simulink model "SMC_PC_Quadcopter_Simulation_SPC_ver2"  (R2013b)
settings: Solver=ode4  StartTime=0.0  StopTime=25  FixedStep=0.02  MaxStep=0.06  RelTol=1e-3
model workspace (MAT data in the model file):
  Sig = Simulink.Signal
  Sig.DataType = 'auto'
  Sig.Dimensions = -1
  Sig.DimensionsMode = 'auto'
  Sig.Complexity = 'auto'
  Sig.SampleTime = -1
  Sig.SamplingMode = 'auto'
undefined symbols (not defined in the file): IC, quadModel
Description:
  | This is a configurable quadcopter simulation.
  | This Simulink model demonstates position control.
  | 
  | Additional quadcopter modeling and simulation materials available at:
  | github.com/dch33/Quad-Sim
  | 
  | Copyright (C) 2014 D. Hartman, K. Landis, S. Moreno, J. Kim, M. Mehrer
  | 
  | License:
  |     This program is free software: you can redistribute it and/or modify
  |     it under the terms of the GNU LESSER GENERAL PUBLIC LICENSE as published by
  |     the Free Software Foundation, either version 3 of the License, or
  |     (at your option) any later version.
  | 
  |     This program is distributed in the hope that it will be useful,
  |     but WITHOUT ANY WARRANTY; without even the implied warranty of
  |     MERCHANTABILITY or FITNESS FOR A PARTICULAR PURPOSE.  See the
  |     GNU General Public License for more details.
  | 
  |     You should have received a copy of the GNU LESSER GENERAL PUBLIC LICENSE
  |     along with this program.  If not, see <http://www.gnu.org/licenses/>.
settings Model: ModifiedComment=SwiftWind -- Mon Apr 06 22:59:35 2015 -- Version 1.6  Creator=David Hartman  LastModifiedBy=SwiftWind
settings Model: ModifiedHistory=|
  | SwiftWind -- Mon Apr 06 22:59:35 2015 -- Version 1.6
  | 
  | 
  | SwiftWind -- Mon Apr 06 22:59:35 2015 -- Version 1.6
  | 
  | 
  | davidhartman -- Fri Jun 06 22:59:54 2014 -- Version 1.5
settings DataIOCC: LimitDataPoints=off  SignalLogging=off
settings OptimizationCC: InlineParams=on
settings DebuggingCC: UnderspecifiedInitializationDetection=Simplified  MergeDetectMultiDrivingBlocksExec=error  UniqueDataStoreMsg=warning  StateNameClashWarn=warning  StrictBusMsg=ErrorOnBusTreatedAsVector

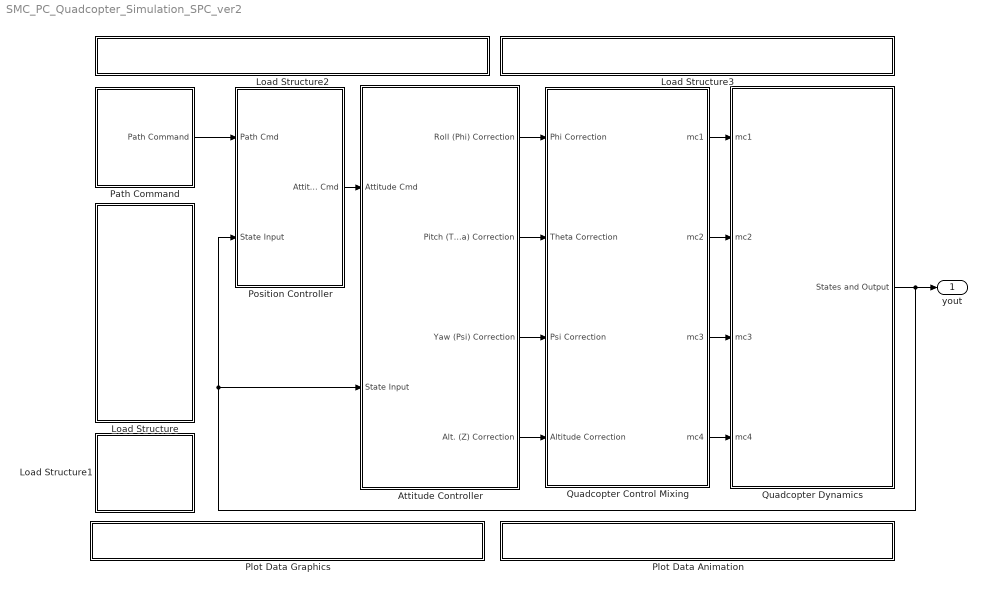
== system SMC_PC_Quadcopter_Simulation_SPC_ver2 ==
  Attitude Controller : Subsystem
  Load Structure : Subsystem
      settings: OpenFcn=|
      | uiopen('load')
      | if ((exist('IC')==1) && (exist('quadModel')==1) && (exist('path')==1))
      | set_param(bdroot, 'SimulationCommand', 'update')
      | end
      mask Display: fprintf('LOAD:\nTimeseries\nPath\nCommands,\nQuadcopter\nModel, Or\nInitial\nConditions');
  Load Structure1 : Subsystem
      settings: OpenFcn=|
      | if (exist('IC')==1 && exist('quadModel')==1 && exist('yout') && exist('tout'))
      | saveSimResults()
      | else
      | msgbox('No Data To Save!')
      | end
      mask Display: fprintf('SAVE:\nSimulation\nResults');
  Load Structure2 : Subsystem
      settings: OpenFcn=|
      | if exist('GUI_Modeling') == 2,
      | run('GUI_Modeling')
      | 
      | else
      | 
      | msgbox('The desired GUI must be first added to MATLABs path.')
      | 
      | end
      mask Display: fprintf('OPEN GUI: Build New \n Model');
  Load Structure3 : Subsystem
      settings: OpenFcn=|
      | if exist('GUI_IC') == 2,
      | run('GUI_IC')
      | 
      | else
      | 
      | msgbox('The desired GUI must be first added to MATLABs path.')
      | 
      | end
      mask Display: fprintf('OPEN GUI: Create Initial \n Conditions');
  Path Command : Subsystem  mask{Interpolate=on, OutputAfterFinalValue=Holding final value}
      mask prompts: Interpolate "Interpolate X, Y, Z, and Psi command data?"; OutputAfterFinalValue "Form output after final data value by:"
      mask help:
      | Selecting the Interpolate data checkbox causes position commands to be
      | linearly interpolated. For additional options related to the Timeseries
      | "path" commands, look under the block and click on the Timeseries From
      | Workspace blocks.
      mask TypeOptions Interpolate: X Timeseries From Wkspace/Interpolate | Y Timeseries From Wkspace/Interpolate | Z Timeseries From Wkspace/Interpolate | Psi Timeseries From Wkspace/Interpolate
      mask TypeOptions OutputAfterFinalValue: X Timeseries From Wkspace/OutputAfterFinalValue | Y Timeseries From Wkspace/OutputAfterFinalValue | Z Timeseries From Wkspace/OutputAfterFinalValue | Psi Timeseries From Wkspace/OutputAfterFinalValue
  Plot Data Animation : Subsystem
      settings: OpenFcn=|
      | if exist('QuadAnim4') == 2,
      |     if exist('yout')
      | 	run('QuadAnim4');
      |     else
      |     msgbox('Simulation must be run before data can be plotted.');
      |     end
      | else                                                                          msgbox('The desired GUI must be first added to MATLABs path.')
      | end
      mask Display: fprintf('OPEN GUI: Flight Animation')
  Plot Data Graphics : Subsystem
      settings: OpenFcn=|
      | if exist('yout')
      | yout = evalin('base', 'yout');
      | tout = evalin('base', 'tout');
      | quadPlots(yout, tout)
      | else
      | msgbox('Simulation must be run before data can be plotted.')
      | end
      mask Display: fprintf('OPEN PLOT: State Data')
  Position Controller : Subsystem
  Quadcopter Control Mixing : Subsystem
      mask Display:
      | modelLoaded = evalin('base','exist(''quadModel'',''var'')');
      | if (modelLoaded==1)
      |     if (evalin('base','quadModel.plusConfig'))
      |     fprintf([' \n' ' \n'  'Configuration "+"']);
      |     else if (~evalin('base','quadModel.plusConfig'))
      |         fprintf([' \n' ' \n' 'Configuration "X"']);
      |         end
      |     end
      | else
      |     fprintf([' \n' ' \n'  'Model Not Loaded']);
      | end
  Quadcopter Dynamics : Subsystem
  yout : Outport
  wires:
  Quadcopter Control Mixing/1(mc1) -> Quadcopter Dynamics/1(mc1)
  Quadcopter Control Mixing/2(mc2) -> Quadcopter Dynamics/2(mc2)
  Quadcopter Control Mixing/3(mc3) -> Quadcopter Dynamics/3(mc3)
  Quadcopter Control Mixing/4(mc4) -> Quadcopter Dynamics/4(mc4)
  Quadcopter Dynamics/1(States and Output) -> yout/1, Attitude Controller/2(State Input), Position Controller/2(State Input)
  Attitude Controller/1(Roll (Phi) Correction) -> Quadcopter Control Mixing/1(Phi Correction)
  Attitude Controller/2(Pitch (Theta) Correction) -> Quadcopter Control Mixing/2(Theta Correction)
  Attitude Controller/3(Yaw (Psi) Correction) -> Quadcopter Control Mixing/3(Psi Correction)
  Attitude Controller/4(Alt. (Z) Correction) -> Quadcopter Control Mixing/4(Altitude Correction)
  Path Command/1("Path Command ") -> Position Controller/1(Path Cmd)
  Position Controller/1(Attitude Cmd) -> Attitude Controller/1(Attitude Cmd)

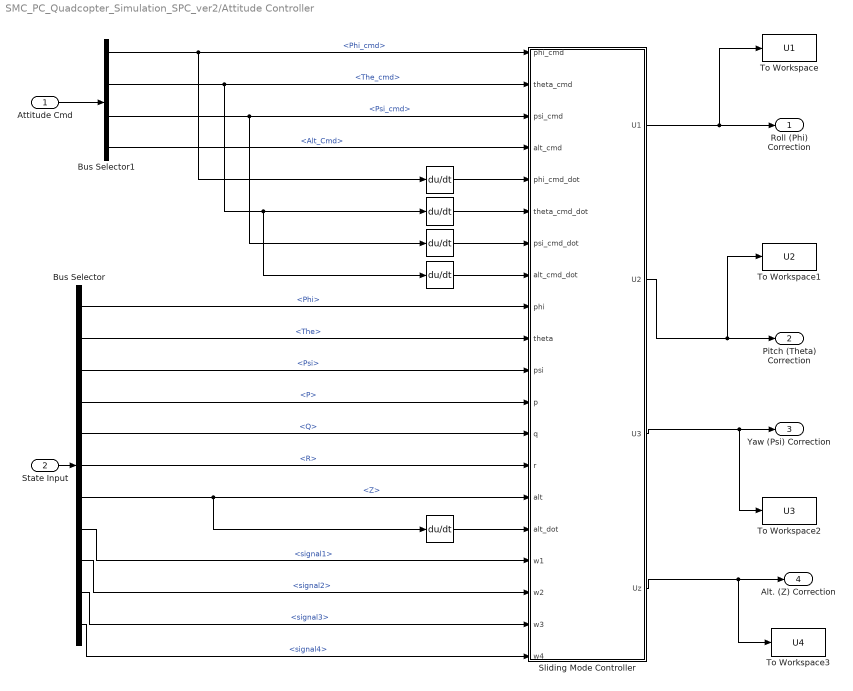
== system SMC_PC_Quadcopter_Simulation_SPC_ver2/Attitude Controller ==
  Attitude Cmd : Inport
  State Input : Inport  Port=2
  " " : Derivative
  " " : Derivative
  "    " : Derivative
  "      " : Derivative
  "        " : Derivative
  Bus Selector : BusSelector  OutputSignals=Phi,The,Psi,P,Q,R,Z,mc and RPM.signal1,mc and RPM.signal2,mc and RPM.signal3,mc and RPM.signal4
  Bus Selector1 : BusSelector  OutputSignals=Phi_cmd,The_cmd,Psi_cmd,Alt_Cmd
  Sliding Mode Controller : MATLAB Function  TreatAsAtomicUnit=on
  To Workspace : ToWorkspace  VariableName=U1  SampleTime=-1  SaveFormat=Timeseries
  To Workspace1 : ToWorkspace  VariableName=U2  SampleTime=-1  SaveFormat=Timeseries
  To Workspace2 : ToWorkspace  VariableName=U3  SampleTime=-1  SaveFormat=Timeseries
  To Workspace3 : ToWorkspace  VariableName=U4  SampleTime=-1  SaveFormat=Timeseries
  Roll (Phi) Correction : Outport
  Pitch (Theta) Correction : Outport  Port=2
  Yaw (Psi) Correction : Outport  Port=3
  Alt. (Z) Correction : Outport  Port=4
  wires:
  Bus Selector/6 -> Sliding Mode Controller/14(r)  "<R>"
  Bus Selector/5 -> Sliding Mode Controller/13(q)  "<Q>"
  Bus Selector/2 -> Sliding Mode Controller/10(theta)  "<The>"
  Bus Selector/3 -> Sliding Mode Controller/11(psi)  "<Psi>"
  State Input/1 -> Bus Selector/1
  Bus Selector/8 -> Sliding Mode Controller/17(w1)  "<signal1>"
  Bus Selector/9 -> Sliding Mode Controller/18(w2)  "<signal2>"
  Bus Selector/10 -> Sliding Mode Controller/19(w3)  "<signal3>"
  Bus Selector/11 -> Sliding Mode Controller/20(w4)  "<signal4>"
  Bus Selector/1 -> Sliding Mode Controller/9(phi)  "<Phi>"
  Bus Selector/7 -> Sliding Mode Controller/15(alt), "        "/1  "<Z>"
  Bus Selector/4 -> Sliding Mode Controller/12(p)  "<P>"
  Attitude Cmd/1 -> Bus Selector1/1
  Bus Selector1/1 -> Sliding Mode Controller/1(phi_cmd), " "/1  "<Phi_cmd>"
  Bus Selector1/2 -> " "/1, "      "/1, Sliding Mode Controller/2(theta_cmd)  "<The_cmd>"
  Bus Selector1/3 -> "    "/1, Sliding Mode Controller/3(psi_cmd)  "<Psi_cmd>"
  Bus Selector1/4 -> Sliding Mode Controller/4(alt_cmd)  "<Alt_Cmd>"
  " "/1 -> Sliding Mode Controller/5(phi_cmd_dot)
  " "/1 -> Sliding Mode Controller/6(theta_cmd_dot)
  "    "/1 -> Sliding Mode Controller/7(psi_cmd_dot)
  "      "/1 -> Sliding Mode Controller/8(alt_cmd_dot)
  Sliding Mode Controller/4(Uz) -> To Workspace3/1, Alt. (Z) Correction/1
  Sliding Mode Controller/1(U1) -> To Workspace/1, Roll (Phi) Correction/1
  Sliding Mode Controller/2(U2) -> To Workspace1/1, Pitch (Theta) Correction/1
  Sliding Mode Controller/3(U3) -> Yaw (Psi) Correction/1, To Workspace2/1
  "        "/1 -> Sliding Mode Controller/16(alt_dot)

== system SMC_PC_Quadcopter_Simulation_SPC_ver2/Load Structure ==

== system SMC_PC_Quadcopter_Simulation_SPC_ver2/Load Structure1 ==

== system SMC_PC_Quadcopter_Simulation_SPC_ver2/Load Structure2 ==

== system SMC_PC_Quadcopter_Simulation_SPC_ver2/Load Structure3 ==

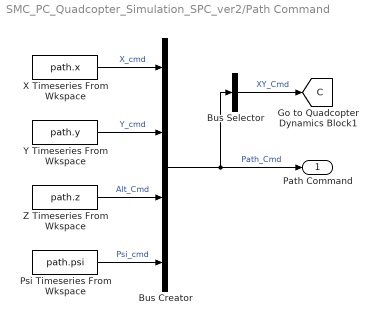
== system SMC_PC_Quadcopter_Simulation_SPC_ver2/Path Command ==
  Bus Creator : BusCreator
  Bus Selector : BusSelector  OutputSignals=X_cmd,Y_cmd  OutputAsBus=on
  Psi Timeseries From Wkspace : FromWorkspace  VariableName=path.psi  SampleTime=0  OutputAfterFinalValue=Holding final value
  X Timeseries From Wkspace : FromWorkspace  VariableName=path.x  SampleTime=0  OutputAfterFinalValue=Holding final value
  Y Timeseries From Wkspace : FromWorkspace  VariableName=path.y  SampleTime=0  OutputAfterFinalValue=Holding final value
  Z Timeseries From Wkspace : FromWorkspace  VariableName=path.z  SampleTime=0  OutputAfterFinalValue=Holding final value
  "Path Command " : Outport
  tag scope: C=global
  wires:
  X Timeseries From Wkspace/1 -> Bus Creator/1  "X_cmd"
  Y Timeseries From Wkspace/1 -> Bus Creator/2  "Y_cmd"
  Z Timeseries From Wkspace/1 -> Bus Creator/3  "Alt_Cmd"
  Psi Timeseries From Wkspace/1 -> Bus Creator/4  "Psi_cmd"
  Bus Creator/1 -> Bus Selector/1, "Path Command "/1  "Path_Cmd"
  Bus Selector/1 -> [C]  "XY_Cmd"

== system SMC_PC_Quadcopter_Simulation_SPC_ver2/Plot Data Animation ==

== system SMC_PC_Quadcopter_Simulation_SPC_ver2/Plot Data Graphics ==

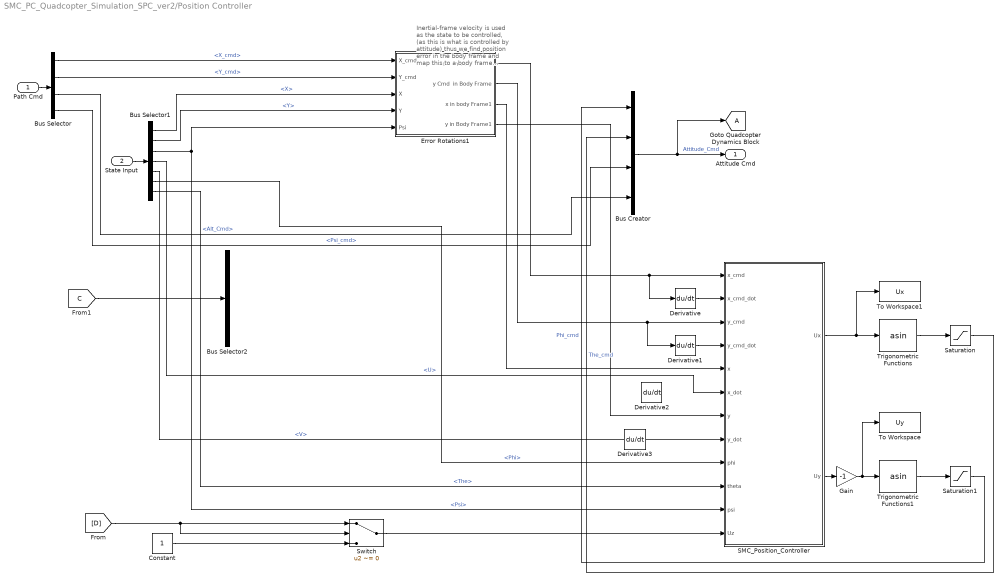
== system SMC_PC_Quadcopter_Simulation_SPC_ver2/Position Controller ==
  note: Inertial-frame velocity is used as the state to be controlled,
      | (as this is what is controlled by attitude)
      | thus we find position error in the body frame
      | and map this to a body frame desired velocity. This desired
      | velocity is then mapped to a desired attitude.
  Path Cmd : Inport
  State Input : Inport  Port=2
  Bus Creator : BusCreator
  Bus Selector : BusSelector  OutputSignals=X_cmd,Y_cmd,Alt_Cmd,Psi_cmd
  Bus Selector1 : BusSelector  OutputSignals=X,Y,Psi,U,V,Phi,The
  Bus Selector2 : BusSelector  OutputSignals=X_cmd,Y_cmd
  Constant : Constant
  Derivative{,1..3} (4 alike) : Derivative
  Error Rotations1 : Subsystem
  Gain : Gain  Gain=-1
  SMC_Position_Controller : MATLAB Function  TreatAsAtomicUnit=on
  Saturation : Saturate  UpperLimit=20*pi/180  LowerLimit=-20*pi/180
  Saturation1 : Saturate  UpperLimit=20*pi/180  LowerLimit=-20*pi/180
  Switch : Switch  Criteria=u2 ~= 0
  To Workspace : ToWorkspace  VariableName=Uy  SampleTime=-1  SaveFormat=Timeseries
  To Workspace1 : ToWorkspace  VariableName=Ux  SampleTime=-1  SaveFormat=Timeseries
  Trigonometric Functions : Trigonometry  Operator=asin
  Trigonometric Functions1 : Trigonometry  Operator=asin
  Attitude Cmd : Outport
  tag scope: A=global
  wires:
  Bus Selector1/5 -> SMC_Position_Controller/8(y_dot)  "<V>"
  State Input/1 -> Bus Selector1/1
  Bus Selector/4 -> Bus Creator/3  "<Psi_cmd>"
  Path Cmd/1 -> Bus Selector/1
  Bus Selector/3 -> Bus Creator/4  "<Alt_Cmd>"
  Bus Creator/1 -> Attitude Cmd/1, [A]  "Attitude_Cmd"
  Bus Selector/1 -> Error Rotations1/1(X_cmd)  "<X_cmd>"
  Bus Selector/2 -> Error Rotations1/2(Y_cmd)  "<Y_cmd>"
  Bus Selector1/1 -> Error Rotations1/3(X)  "<X>"
  Bus Selector1/2 -> Error Rotations1/4(Y)  "<Y>"
  Bus Selector1/3 -> Error Rotations1/5(Psi), SMC_Position_Controller/11(psi)  "<Psi>"
  Bus Selector1/4 -> SMC_Position_Controller/6(x_dot)  "<U>"
  [C] -> Bus Selector2/1
  Derivative/1 -> SMC_Position_Controller/2(x_cmd_dot)
  Derivative1/1 -> SMC_Position_Controller/4(y_cmd_dot)
  Bus Selector1/6 -> SMC_Position_Controller/9(phi)  "<Phi>"
  Bus Selector1/7 -> SMC_Position_Controller/10(theta)  "<The>"
  SMC_Position_Controller/1(Ux) -> To Workspace1/1, Trigonometric Functions/1
  [D] -> Switch/2, Switch/1
  Constant/1 -> Switch/3
  Switch/1 -> SMC_Position_Controller/12(Uz)
  Trigonometric Functions/1 -> Saturation/1
  Trigonometric Functions1/1 -> Saturation1/1
  Saturation1/1 -> Bus Creator/1  "Phi_cmd"
  Saturation/1 -> Bus Creator/2  "The_cmd"
  Error Rotations1/1(x Cmd  in body Frame) -> Derivative/1, SMC_Position_Controller/1(x_cmd)
  Error Rotations1/2(y Cmd  in Body Frame) -> Derivative1/1, SMC_Position_Controller/3(y_cmd)
  Error Rotations1/3(x in body Frame1) -> SMC_Position_Controller/5(x)
  Error Rotations1/4(y in Body Frame1) -> SMC_Position_Controller/7(y)
  SMC_Position_Controller/2(Uy) -> Gain/1
  Gain/1 -> To Workspace/1, Trigonometric Functions1/1

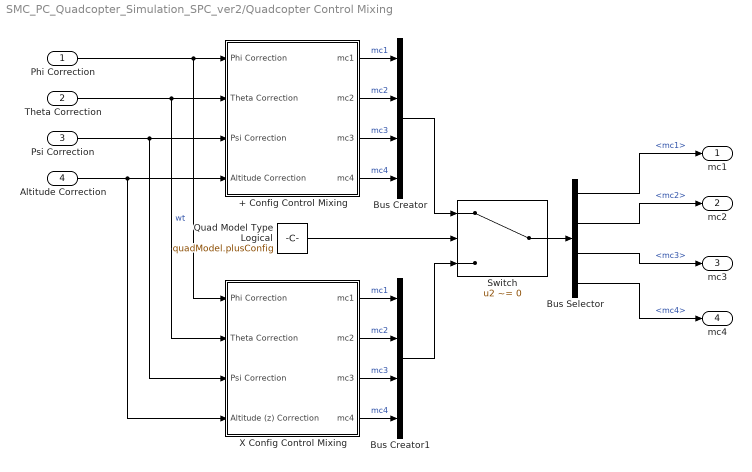
== system SMC_PC_Quadcopter_Simulation_SPC_ver2/Quadcopter Control Mixing ==
  Phi Correction : Inport
  Theta Correction : Inport  Port=2
  Psi Correction : Inport  Port=3
  Altitude Correction : Inport  Port=4
  + Config Control Mixing : Subsystem
  Bus Creator : BusCreator
  Bus Creator1 : BusCreator
  Bus Selector : BusSelector  OutputSignals=mc1,mc2,mc3,mc4
  Quad Model Type Logical : Constant  Value=quadModel.plusConfig
  Switch : Switch  Criteria=u2 ~= 0
  X Config Control Mixing : Subsystem
  mc1 : Outport
  mc2 : Outport  Port=2
  mc3 : Outport  Port=3
  mc4 : Outport  Port=4
  wires:
  Phi Correction/1 -> X Config Control Mixing/1(Phi Correction), + Config Control Mixing/1(Phi Correction)
  Theta Correction/1 -> X Config Control Mixing/2(Theta Correction), + Config Control Mixing/2(Theta Correction)  "wt"
  Psi Correction/1 -> X Config Control Mixing/3(Psi Correction), + Config Control Mixing/3(Psi Correction)
  Altitude Correction/1 -> X Config Control Mixing/4(Altitude (z) Correction), + Config Control Mixing/4(Altitude Correction)
  + Config Control Mixing/1(mc1) -> Bus Creator/1  "mc1"
  + Config Control Mixing/2(mc2) -> Bus Creator/2  "mc2"
  + Config Control Mixing/3(mc3) -> Bus Creator/3  "mc3"
  + Config Control Mixing/4(mc4) -> Bus Creator/4  "mc4"
  Bus Creator/1 -> Switch/1
  X Config Control Mixing/1(mc1) -> Bus Creator1/1  "mc1"
  X Config Control Mixing/2(mc2) -> Bus Creator1/2  "mc2"
  X Config Control Mixing/3(mc3) -> Bus Creator1/3  "mc3"
  X Config Control Mixing/4(mc4) -> Bus Creator1/4  "mc4"
  Bus Creator1/1 -> Switch/3
  Bus Selector/1 -> mc1/1  "<mc1>"
  Bus Selector/2 -> mc2/1  "<mc2>"
  Bus Selector/3 -> mc3/1  "<mc3>"
  Bus Selector/4 -> mc4/1  "<mc4>"
  Quad Model Type Logical/1 -> Switch/2
  Switch/1 -> Bus Selector/1

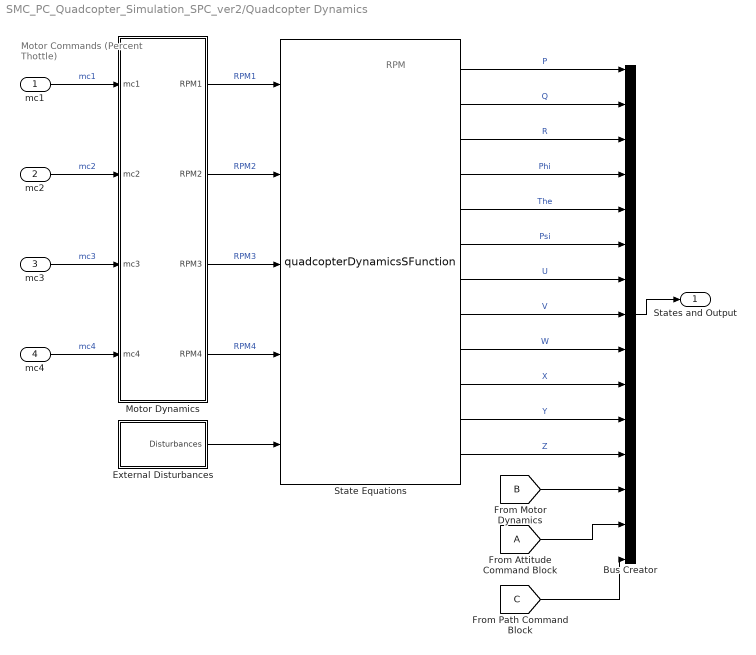
== system SMC_PC_Quadcopter_Simulation_SPC_ver2/Quadcopter Dynamics ==
  note: RPM
  note: Motor Commands
      | (Percent Thottle)
  mc1 : Inport
  mc2 : Inport  Port=2
  mc3 : Inport  Port=3
  mc4 : Inport  Port=4
  Bus Creator : BusCreator  Inputs='P','Q','R','Phi','The','Psi','U','V','W','X','Y','Z','mc and RPM','Attitude_Cmd','XY_Cmd'
  External Disturbances : Subsystem
  Motor Dynamics : Subsystem
  State Equations : M-S-Function  FunctionName=quadcopterDynamicsSFunction  Parameters=quadModel, IC
      mask Display:
      | port_label('input', 1, 'RPM1')
      | port_label('input', 2, 'RPM2')
      | port_label('input', 3, 'RPM3')
      | port_label('input', 4, 'RPM4')
      | port_label('input', 5, 'Disturbances')
      | port_label('output', 1, 'P')
      | port_label('output', 2, 'Q')
      | port_label('output', 3, 'R')
      | port_label('output', 4, 'Phi')
      | port_label('output', 5, 'The')
      | port_label('output', 6, 'Psi')
      | port_label('output', 7, 'U')
      | port_label('output', 8, 'V')
      | port_label('output', 9, 'W')
      | port_label('output', 10, 'X')
      | port_label('output', 11, 'Y')
      | port_label('output', 12, 'Z')
  States and Output : Outport
  wires:
  State Equations/1 -> Bus Creator/1  "P"
  State Equations/2 -> Bus Creator/2  "Q"
  State Equations/3 -> Bus Creator/3  "R"
  State Equations/4 -> Bus Creator/4  "Phi"
  State Equations/5 -> Bus Creator/5  "The"
  State Equations/6 -> Bus Creator/6  "Psi"
  State Equations/7 -> Bus Creator/7  "U"
  State Equations/8 -> Bus Creator/8  "V"
  State Equations/9 -> Bus Creator/9  "W"
  State Equations/10 -> Bus Creator/10  "X"
  State Equations/11 -> Bus Creator/11  "Y"
  State Equations/12 -> Bus Creator/12  "Z"
  Bus Creator/1 -> States and Output/1
  Motor Dynamics/1(RPM1) -> State Equations/1  "RPM1"
  Motor Dynamics/2(RPM2) -> State Equations/2  "RPM2"
  Motor Dynamics/3(RPM3) -> State Equations/3  "RPM3"
  Motor Dynamics/4(RPM4) -> State Equations/4  "RPM4"
  mc1/1 -> Motor Dynamics/1(mc1)  "mc1"
  mc4/1 -> Motor Dynamics/4(mc4)  "mc4"
  mc3/1 -> Motor Dynamics/3(mc3)  "mc3"
  mc2/1 -> Motor Dynamics/2(mc2)  "mc2"
  External Disturbances/1("Disturbances ") -> State Equations/5
  [A] -> Bus Creator/14
  [B] -> Bus Creator/13
  [C] -> Bus Creator/15

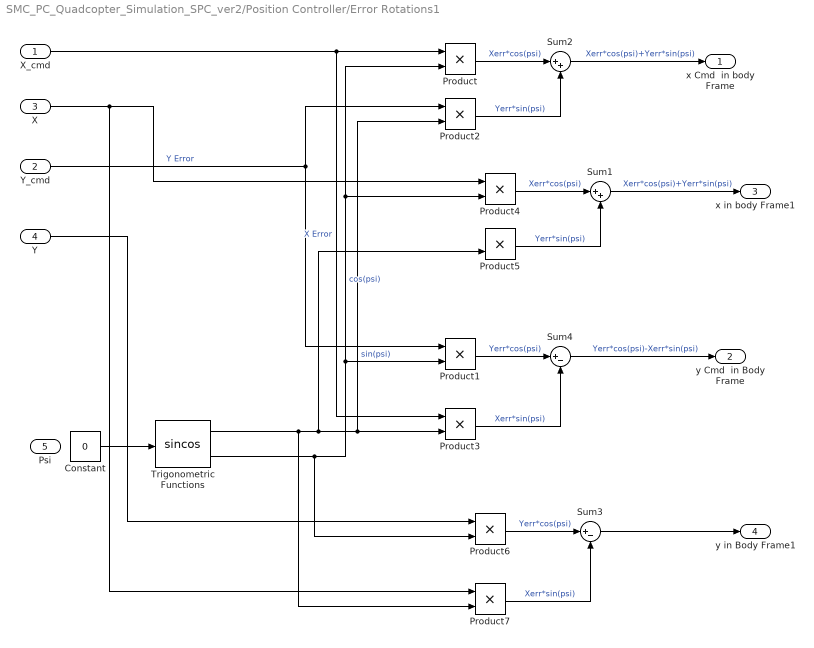
== system SMC_PC_Quadcopter_Simulation_SPC_ver2/Position Controller/Error Rotations1 ==
  X_cmd : Inport
  Y_cmd : Inport  Port=2
  X : Inport  Port=3
  Y : Inport  Port=4
  Psi : Inport  Port=5
  Constant : Constant  Value=0
  Product{,1..7} (8 alike) : Product
  Sum1 : Sum  Inputs=|++
  Sum2 : Sum  Inputs=|++
  Sum3 : Sum  Inputs=|+-
  Sum4 : Sum  Inputs=|+-
  Trigonometric Functions : Trigonometry  Operator=sincos
  x Cmd  in body Frame : Outport
  y Cmd  in Body Frame : Outport  Port=2
  x in body Frame1 : Outport  Port=3
  y in Body Frame1 : Outport  Port=4
  wires:
  Product1/1 -> Sum4/1  "Yerr*cos(psi)"
  Product2/1 -> Sum2/2  "Yerr*sin(psi)"
  Product/1 -> Sum2/1  "Xerr*cos(psi)"
  Trigonometric Functions/2 -> Product6/2, Product1/2, Product/2, Product4/2  "cos(psi)"
  X_cmd/1 -> Product/1, Product3/1  "X Error"
  Y/1 -> Product6/1
  Sum2/1 -> x Cmd  in body Frame/1  "Xerr*cos(psi)+Yerr*sin(psi)"
  Trigonometric Functions/1 -> Product7/2, Product5/2, Product3/2, Product2/2  "sin(psi)"
  Y_cmd/1 -> Product1/1, Product2/1  "Y Error"
  Product3/1 -> Sum4/2  "Xerr*sin(psi)"
  Sum4/1 -> y Cmd  in Body Frame/1  "Yerr*cos(psi)-Xerr*sin(psi)"
  Product5/1 -> Sum1/2  "Yerr*sin(psi)"
  Product4/1 -> Sum1/1  "Xerr*cos(psi)"
  Sum1/1 -> x in body Frame1/1  "Xerr*cos(psi)+Yerr*sin(psi)"
  X/1 -> Product7/1, Product4/1
  Product6/1 -> Sum3/1  "Yerr*cos(psi)"
  Product7/1 -> Sum3/2  "Xerr*sin(psi)"
  Sum3/1 -> y in Body Frame1/1
  Constant/1 -> Trigonometric Functions/1

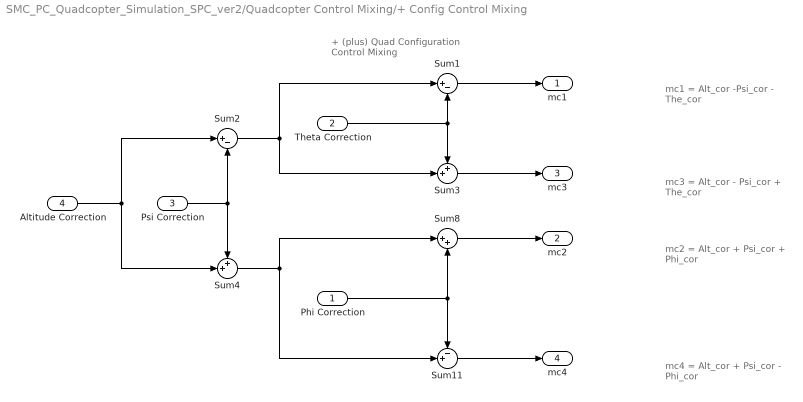
== system SMC_PC_Quadcopter_Simulation_SPC_ver2/Quadcopter Control Mixing/+ Config Control Mixing ==
  note: mc2 = Alt_cor + Psi_cor + Phi_cor
  note: + (plus) Quad Configuration Control Mixing
  note: mc4 = Alt_cor + Psi_cor - Phi_cor
  note: mc3 = Alt_cor - Psi_cor + The_cor
  note: mc1 = Alt_cor -Psi_cor - The_cor
  Phi Correction : Inport
  Theta Correction : Inport  Port=2
  Psi Correction : Inport  Port=3
  Altitude Correction : Inport  Port=4
  Sum1 : Sum  Inputs=|+-
  Sum11 : Sum  Inputs=-+|
  Sum2 : Sum  Inputs=|+-
  Sum3 : Sum  Inputs=++|
  Sum4 : Sum  Inputs=++|
  Sum8 : Sum  Inputs=|++
  mc1 : Outport
  mc2 : Outport  Port=2
  mc3 : Outport  Port=3
  mc4 : Outport  Port=4
  wires:
  Theta Correction/1 -> Sum1/2, Sum3/1
  Altitude Correction/1 -> Sum2/1, Sum4/2
  Sum2/1 -> Sum3/2, Sum1/1
  Psi Correction/1 -> Sum4/1, Sum2/2
  Sum4/1 -> Sum11/2, Sum8/1
  Phi Correction/1 -> Sum8/2, Sum11/1
  Sum1/1 -> mc1/1
  Sum3/1 -> mc3/1
  Sum8/1 -> mc2/1
  Sum11/1 -> mc4/1

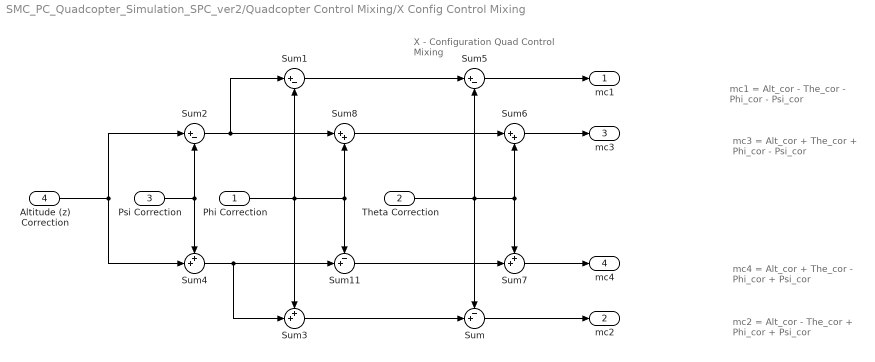
== system SMC_PC_Quadcopter_Simulation_SPC_ver2/Quadcopter Control Mixing/X Config Control Mixing ==
  note: mc1 = Alt_cor - The_cor - Phi_cor - Psi_cor
  note: X - Configuration Quad Control Mixing
  note: mc3 = Alt_cor + The_cor + Phi_cor - Psi_cor
  note: mc2 = Alt_cor - The_cor + Phi_cor + Psi_cor
  note: mc4 = Alt_cor + The_cor - Phi_cor + Psi_cor
  Phi Correction : Inport
  Theta Correction : Inport  Port=2
  Psi Correction : Inport  Port=3
  Altitude (z) Correction : Inport  Port=4
  Sum : Sum  Inputs=-+|
  Sum1 : Sum  Inputs=|+-
  Sum11 : Sum  Inputs=-+|
  Sum2 : Sum  Inputs=|+-
  Sum3 : Sum  Inputs=++|
  Sum4 : Sum  Inputs=++|
  Sum5 : Sum  Inputs=|+-
  Sum6 : Sum  Inputs=|++
  Sum7 : Sum  Inputs=++|
  Sum8 : Sum  Inputs=|++
  mc1 : Outport
  mc2 : Outport  Port=2
  mc3 : Outport  Port=3
  mc4 : Outport  Port=4
  wires:
  Sum2/1 -> Sum8/1, Sum1/1
  Psi Correction/1 -> Sum4/1, Sum2/2
  Phi Correction/1 -> Sum3/1, Sum1/2, Sum8/2, Sum11/1
  Sum4/1 -> Sum3/2, Sum11/2
  Sum3/1 -> Sum/2
  Theta Correction/1 -> Sum7/1, Sum6/2, Sum5/2, Sum/1
  Sum1/1 -> Sum5/1
  Sum8/1 -> Sum6/1
  Sum11/1 -> Sum7/2
  Sum5/1 -> mc1/1
  Sum6/1 -> mc3/1
  Sum7/1 -> mc4/1
  Altitude (z) Correction/1 -> Sum2/1, Sum4/2
  Sum/1 -> mc2/1

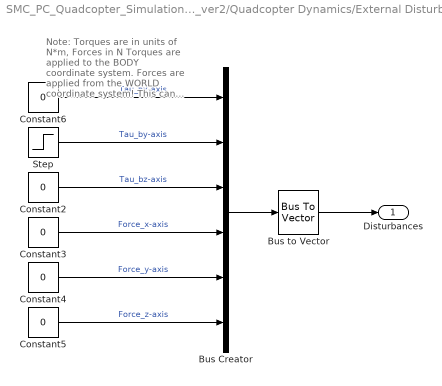
== system SMC_PC_Quadcopter_Simulation_SPC_ver2/Quadcopter Dynamics/External Disturbances ==
  note: Note: Torques are in units of N*m, Forces in N
      | Torques are applied to the BODY coordinate system.
      | Forces are applied from the WORLD coordinate system!
      | This can be changed by adjusting the equations within the S-function.
  Bus Creator : BusCreator  Inputs=6
  Bus to Vector : BusToVector
  Constant{2..6} (5 alike) : Constant  Value=0
  Step : Step  After=0  SampleTime=0
  "Disturbances " : Outport
  wires:
  Bus to Vector/1 -> "Disturbances "/1
  Bus Creator/1 -> Bus to Vector/1
  Constant6/1 -> Bus Creator/1  "Tau_bx-axis"
  Step/1 -> Bus Creator/2  "Tau_by-axis"
  Constant2/1 -> Bus Creator/3  "Tau_bz-axis"
  Constant3/1 -> Bus Creator/4  "Force_x-axis"
  Constant4/1 -> Bus Creator/5  "Force_y-axis"
  Constant5/1 -> Bus Creator/6  "Force_z-axis"

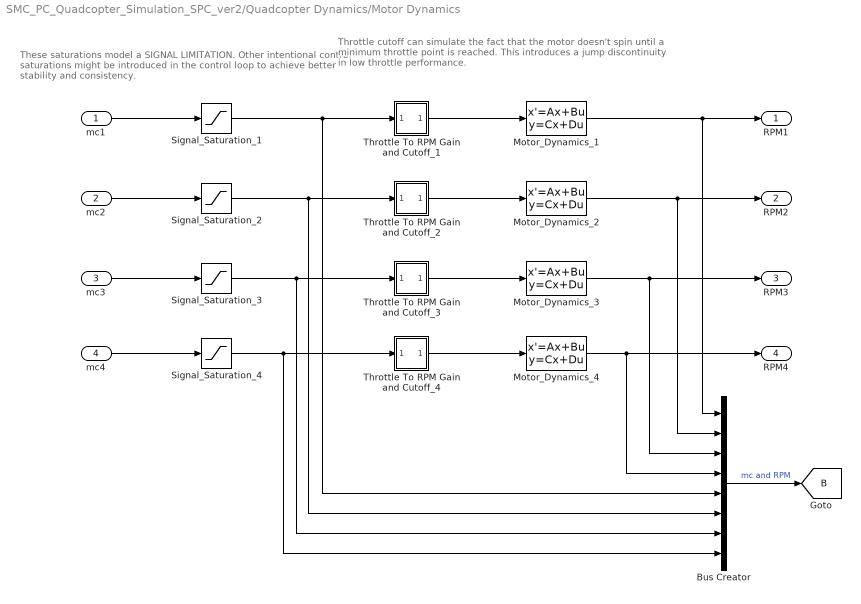
== system SMC_PC_Quadcopter_Simulation_SPC_ver2/Quadcopter Dynamics/Motor Dynamics ==
  note: These saturations model a SIGNAL LIMITATION.
      | Other intentional control saturations might be introduced in the
      | control loop to achieve better stability and consistency.
  note: Throttle cutoff can simulate the fact that the motor doesn't
      | spin until a minimum throttle point is reached. This introduces
      | a jump discontinuity in low throttle performance.
  mc1 : Inport
  mc2 : Inport  Port=2
  mc3 : Inport  Port=3
  mc4 : Inport  Port=4
  Bus Creator : BusCreator  Inputs=8
  Motor_Dynamics_1 : StateSpace  A=-1/quadModel.T  C=1/quadModel.T  D=0  X0=IC.w1*quadModel.T
  Motor_Dynamics_2 : StateSpace  A=-1/quadModel.T  C=1/quadModel.T  D=0  X0=IC.w2*quadModel.T
  Motor_Dynamics_3 : StateSpace  A=-1/quadModel.T  C=1/quadModel.T  D=0  X0=IC.w3*quadModel.T
  Motor_Dynamics_4 : StateSpace  A=-1/quadModel.T  C=1/quadModel.T  D=0  X0=IC.w4*quadModel.T
  Signal_Saturation_{1..4} (4 alike) : Saturate  UpperLimit=100  LowerLimit=0
  Throttle To RPM Gain and Cutoff_1 : Subsystem
  Throttle To RPM Gain and Cutoff_2 : Subsystem
  Throttle To RPM Gain and Cutoff_3 : Subsystem
  Throttle To RPM Gain and Cutoff_4 : Subsystem
  RPM1 : Outport
  RPM2 : Outport  Port=2
  RPM3 : Outport  Port=3
  RPM4 : Outport  Port=4
  tag scope: B=global
  wires:
  Bus Creator/1 -> [B]  "mc and RPM"
  Motor_Dynamics_4/1 -> RPM4/1, Bus Creator/4
  Motor_Dynamics_3/1 -> RPM3/1, Bus Creator/3
  Motor_Dynamics_2/1 -> RPM2/1, Bus Creator/2
  Motor_Dynamics_1/1 -> RPM1/1, Bus Creator/1
  Throttle To RPM Gain and Cutoff_4/1(Out5) -> Motor_Dynamics_4/1
  Throttle To RPM Gain and Cutoff_3/1(Out5) -> Motor_Dynamics_3/1
  Throttle To RPM Gain and Cutoff_2/1(Out5) -> Motor_Dynamics_2/1
  Throttle To RPM Gain and Cutoff_1/1(Out5) -> Motor_Dynamics_1/1
  Signal_Saturation_4/1 -> Throttle To RPM Gain and Cutoff_4/1(In5), Bus Creator/8
  Signal_Saturation_3/1 -> Throttle To RPM Gain and Cutoff_3/1(In5), Bus Creator/7
  Signal_Saturation_2/1 -> Throttle To RPM Gain and Cutoff_2/1(In5), Bus Creator/6
  Signal_Saturation_1/1 -> Throttle To RPM Gain and Cutoff_1/1(In5), Bus Creator/5
  mc3/1 -> Signal_Saturation_3/1
  mc2/1 -> Signal_Saturation_2/1
  mc4/1 -> Signal_Saturation_4/1
  mc1/1 -> Signal_Saturation_1/1

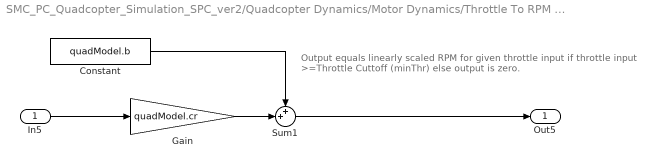
== system SMC_PC_Quadcopter_Simulation_SPC_ver2/Quadcopter Dynamics/Motor Dynamics/Throttle To RPM Gain and Cutoff_1 ==
  note: Output equals linearly scaled RPM
      | for given throttle input if throttle input >=Throttle Cuttoff (minThr)
      | else output is zero.
  In5 : Inport
  Constant : Constant  Value=quadModel.b
  Gain : Gain  Gain=quadModel.cr
  Sum1 : Sum  Inputs=++|
  Out5 : Outport
  wires:
  Constant/1 -> Sum1/1
  Gain/1 -> Sum1/2
  In5/1 -> Gain/1
  Sum1/1 -> Out5/1

== system SMC_PC_Quadcopter_Simulation_SPC_ver2/Quadcopter Dynamics/Motor Dynamics/Throttle To RPM Gain and Cutoff_2 ==
  note: Output equals linearly scaled RPM
      | for given throttle input if throttle input >=Throttle Cuttoff (minThr)
      | else output is zero.
  In5 : Inport
  Constant : Constant  Value=quadModel.b
  Gain : Gain  Gain=quadModel.cr
  Sum1 : Sum  Inputs=++|
  Out5 : Outport
  wires:
  Constant/1 -> Sum1/1
  Gain/1 -> Sum1/2
  In5/1 -> Gain/1
  Sum1/1 -> Out5/1

== system SMC_PC_Quadcopter_Simulation_SPC_ver2/Quadcopter Dynamics/Motor Dynamics/Throttle To RPM Gain and Cutoff_3 ==
  note: Output equals linearly scaled RPM
      | for given throttle input if throttle input >=Throttle Cuttoff (minThr)
      | else output is zero.
  In5 : Inport
  Constant : Constant  Value=quadModel.b
  Gain : Gain  Gain=quadModel.cr
  Sum1 : Sum  Inputs=++|
  Out5 : Outport
  wires:
  Constant/1 -> Sum1/1
  Gain/1 -> Sum1/2
  In5/1 -> Gain/1
  Sum1/1 -> Out5/1

== system SMC_PC_Quadcopter_Simulation_SPC_ver2/Quadcopter Dynamics/Motor Dynamics/Throttle To RPM Gain and Cutoff_4 ==
  note: Output equals linearly scaled RPM
      | for given throttle input if throttle input >=Throttle Cuttoff (minThr)
      | else output is zero.
  In5 : Inport
  Constant : Constant  Value=quadModel.b
  Gain : Gain  Gain=quadModel.cr
  Sum1 : Sum  Inputs=++|
  Out5 : Outport
  wires:
  Constant/1 -> Sum1/1
  Gain/1 -> Sum1/2
  In5/1 -> Gain/1
  Sum1/1 -> Out5/1

== matlab function SMC_PC_Quadcopter_Simulation_SPC_ver2/Position Controller/SMC_Position_Controller ==
  data: x_cmd input; Ux output; x_cmd_dot input; y_cmd input; y_cmd_dot input; x input; x_dot input; y input; y_dot input; phi input; theta input; psi input; Uy output; Uz input
%% Sliding Mode Controller - X,Y Position
function [Ux, Uy] = SMC_Position_xy(x_cmd,x_cmd_dot,y_cmd,y_cmd_dot,x,x_dot,y,y_dot,phi,theta,psi,Uz)
%% SMC Initial Setup
% Retrieve Parameter from Model
% Ix = Model.Jx;
% Iy = Model.Jy;
% Iz = Model.Jz;
Jr = 3.441e-04; % Propeller Inertia Using 2/3*MR^2 [kg*m^2]
% l = Model.arms_L; % Quadrotor CoG to Motor Length

Ix = [0.0132610000000000];
Iy = [0.0132610000000000];
Iz = [0.0253620000000000];
l = 0.25;
m = 1.05;

a1 = (Iy-Iz)/Ix;
a2 = Jr/Ix;
a3 = (Iz-Ix)/Iy;
a4 = Jr/Iy;
a5 = (Ix-Iy)/Iz;


b1 = l/Ix;
b2 = l/Iy;
b3 = 1/Iz;

%% SMC Control Gains

% Inertial Frame Position - X Controller Gains
alpha_x = 0.1;
Kx = [0.1 0.1];

% Inertial Frame Position - Y Controller Gains
alpha_y = 0.1;
Ky = [0.1 0.1];

%% Sliding Surface
% Sliding Surface for Tracking Control 
% % for Roll
% z1 = phi_cmd - phi;
% % z1 = -z1;
% S1 = p - phi_cmd_dot - alpha1*z1; 
% 
% % for Theta
% z2 = theta_cmd - theta;
% % z2 = -z2;
% S2 = q - theta_cmd_dot - alpha2*z2;
% 
% % for Psi
% z3 = psi_cmd - psi;
% % z3 = -z3;
% S3 = r - psi_cmd_dot - alpha3*z3;
% 
% % for Z 
% % zz = alt_cmd - alt;
% % Sz = alt_dot - alt_cmd_dot - alpha_z*zz;

% for x
zx = x_cmd - x;
Sx = x_dot - x_cmd_dot - alpha_x*zx;

% for y
zy = y_cmd - y;
Sy = y_dot - y_cmd_dot - alpha_y*zy;
%% Sliding Controller
% Uz = m/(cos(phi)*cos(theta))*(-Kz(1)*sat(Sz) - Kz(2)*Sz + alpha_z*(alt_cmd_dot - alt_dot) + 9.81);
% Ux = m/Uz*(-Kx(1) * sat(Sx) - Kx(2) * Sx + alpha_x*(x_cmd_dot - x_dot))/(cos(phi)*sin(theta)*cos(psi) + sin(phi)*sin(psi));
% Uy = m/Uz*(-Ky(1) * sat(Sy) - Ky(2) * Sy + alpha_y*(y_cmd_dot - y_dot))/(cos(phi)*sin(theta)*sin(psi) - sin(phi)*sin(psi));
Ux = m/Uz*(-Kx(1) * sat(Sx) - Kx(2) * Sx + alpha_x*(x_cmd_dot - x_dot))/cos(phi);
Uy = m/Uz*(-Ky(1) * sat(Sy) - Ky(2) * Sy + alpha_y*(y_cmd_dot - y_dot));

== matlab function SMC_PC_Quadcopter_Simulation_SPC_ver2/Attitude Controller/Sliding Mode Controller ==
  data: phi_cmd input; theta_cmd input; psi_cmd input; alt_cmd input; phi_cmd_dot input; theta_cmd_dot input; psi_cmd_dot input; alt_cmd_dot input; phi input; theta input; psi input; U1 output; p input; q input; r input; alt input; alt_dot input; w1 input; w2 input; w3 input; w4 input; U2 output; U3 output; Uz output
%% Sliding Mode for Attitude Control of Quadrotor
% z : New State for Tracking Control (Command - Feedback)
function [U1,U2,U3, Uz]  = SMC_Attitude(phi_cmd, theta_cmd, psi_cmd, alt_cmd, phi_cmd_dot, theta_cmd_dot, psi_cmd_dot, alt_cmd_dot, phi, theta, psi, p, q, r, alt, alt_dot,w1, w2, w3, w4)
%% SMC Initial Setup
% Retrieve Parameter from Model
% Ix = Model.Jx;
% Iy = Model.Jy;
% Iz = Model.Jz;
Jr = 3.441e-04; % Propeller Inertia Using 2/3*MR^2 [kg*m^2]
% l = Model.arms_L; % Quadrotor CoG to Motor Length

Ix = 0.012706;
Iy = 0.012706;
Iz = 0.024253;
l = 0.25;
m = 1.05;

a1 = (Iy-Iz)/Ix;
a2 = Jr/Ix;
a3 = (Iz-Ix)/Iy;
a4 = Jr/Iy;
a5 = (Ix-Iy)/Iz;


b1 = l/Ix;
b2 = l/Iy;
b3 = 1/Iz;

OMG_r = (w1 + w3 - w2 - w4) * 2*pi/60; 
% Motors Ang. Vel. Expressing Gyroscopic Forces [rad/s]

%% SMC Control Gains
% Roll Controller Gains
alpha1 = 3;
% K1 = [25 50];
% K1 = [16 8];
K1 = [50 100];
% Pitch Controller Gains
% is same as Roll Control due to Symmetry
alpha2 = 3;
K2 = [50 100];

% Yaw Controller Gains
alpha3 = 5;
K3 = [100 50];

% Altitude Controller Gains
alpha_z = 5;
Kz = [20 3];

% % SMC Control Gains
% Roll Controller Gains
% alpha1 = 2;
% K1 = [30 15];
% K1 = [16 8];
% K1 = [10 5];
% Pitch Controller Gains
% is same as Roll Control due to Symmetry
% alpha2 = alpha1;
% K2 = K1;
% 
% Yaw Controller Gains
% alpha3 = 2;
% K3 = [30 15];
% 
% Altitude Controller Gains
% alpha_z = 5;
% Kz = [20 3];

%% Sliding Surface
% Sliding Surface for Tracking Control 
% for Roll
z1 = phi_cmd - phi;
% z1 = -z1;
S1 = p - phi_cmd_dot - alpha1*z1; 

% for Theta
z2 = theta_cmd - theta;
% z2 = -z2;
S2 = q - theta_cmd_dot - alpha2*z2;

% for Psi
z3 = psi_cmd - psi;
% z3 = -z3;
S3 = r - psi_cmd_dot - alpha3*z3;

% for Z 
zz = alt_cmd - alt;
Sz = alt_dot - alt_cmd_dot - alpha_z*zz;

%% Sliding Controller
% a2 = 0; a4 =0;
% Boudallah Thesis Sliding by Backstepping Approach
% U1 = 1/b1*(-a1*q*r - a2*q*OMG_r - alpha1^2*z1 - K1(1)*sat(S1) - K1(2)*S1);
% 
% U2 = 1/b2*(a3*p*r - a4*p*OMG_r - alpha2^2*z2 - K2(1)*sat(S2) - K2(2)*S2);
% 
% U3 = 1/b3*(-a5*p*q - alpha3^2*z3 - K3(1)*sat(S3) - K3(2)*S3);

% Bouadi Paper Sliding Control by Backstepping Approach
U1 = 1/b1*(-a1*q*r + a2*OMG_r*q - K1(1)*sat(S1) - K1(2)*S1 + alpha1*(phi_cmd_dot - p));
U2 = 1/b2*(-a3*p*r - a4*p*OMG_r +alpha2*(theta_cmd_dot - q) -K2(1)*sat(S2) - K2(2)*S2);
U3 = 1/b3*(-a5*p*q - K3(1)*sat(S3) - K3(2)*S3 + alpha3*(psi_cmd_dot-r));
Uz = m/(cos(phi)*cos(theta))*(-Kz(1)*sat(Sz) - Kz(2)*Sz + alpha_z*(alt_cmd_dot - alt_dot) + 9.81);
